simulink model "fig4_21sim"  (Simulink 7.9)
settings: Solver=ode45  SolverMode=SingleTasking  StartTime=0.0  StopTime=5  RelTol=1e-3  AbsTol=1e-6
undefined symbols (not defined in the file or in its folder): denD, numD, T
libraries: simulink x2
settings Model: Creator=Gene Franklin  LastModifiedBy=abbas  ExtModeTrigMode=oneshot  ExtModeArmWhenConnect=off
settings DataIOCC: LimitDataPoints=off
settings OptimizationCC: BlockReduction=off  BooleanDataType=off
settings DebuggingCC: SaveWithParameterizedLinksMsg=none  SignalResolutionControl=TryResolveAllWithWarning  SolverPrmCheckMsg=none  MultiTaskDSMMsg=warning  MultiTaskCondExecSysMsg=none  FcnCallInpInsideContextMsg=Use local settings  StrictBusMsg=None
settings HardwareCC: TargetUnknown=on
settings RTWCC: IncludeERTFirstTime=on
settings GRTTargetCC: CombineOutputUpdateFcns=off  GRTInterface=on

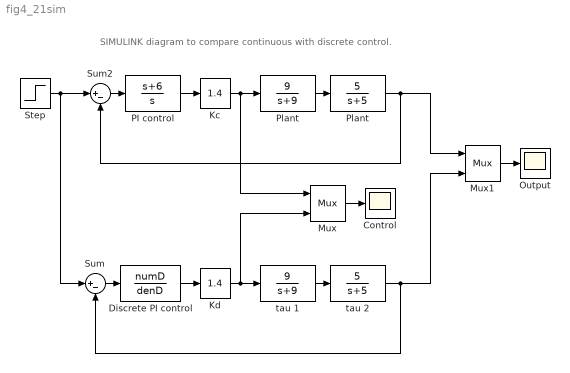
== system fig4_21sim ==
  note: SIMULINK diagram to compare continuous with discrete control.
  Control : Scope
      settings: TickLabels=on  YMin=0  YMax=2.75  SaveName=ucd
  Discrete PI control : DiscreteTransferFcn  Numerator=numD  Denominator=denD  SampleTime=T
  Kc : simulink/Math Operations/Slider Gain  low=0  gain=1.4  high=10
  Kd : simulink/Math Operations/Slider Gain  low=0  gain=1.4  high=10
  Mux : Mux  Inputs=2
  Mux1 : Mux  Inputs=2
  Output : Scope
      settings: TickLabels=on  SaveName=ycd
  PI control : TransferFcn  Numerator=[1 6]  Denominator=[1 0]
  Plant : TransferFcn  Numerator=[9]  Denominator=[1 9]
  "Plant " : TransferFcn  Numerator=[5]  Denominator=[1 5]
  Step : Step  Time=.1  SampleTime=.001
  Sum : Sum  Inputs=|+-  InputSameDT=on  OutDataTypeStr=Inherit: Same as first input
  Sum2 : Sum  Inputs=|+-  InputSameDT=on  OutDataTypeStr=Inherit: Same as first input
  tau 1 : TransferFcn  Numerator=[9]  Denominator=[1 9]
  tau 2 : TransferFcn  Numerator=[5]  Denominator=[1 5]
  wires:
  PI control/1 -> Kc/1
  Sum2/1 -> PI control/1
  Plant/1 -> "Plant "/1
  Discrete PI control/1 -> Kd/1
  tau 1/1 -> tau 2/1
  Step/1 -> Sum2/1, Sum/1
  Kc/1 -> Plant/1, Mux/1
  Mux/1 -> Control/1
  "Plant "/1 -> Mux1/1, Sum2/2
  Mux1/1 -> Output/1
  Sum/1 -> Discrete PI control/1
  Kd/1 -> tau 1/1, Mux/2
  tau 2/1 -> Mux1/2, Sum/2
